simulink model "W3prob2"  (R2020b)
settings: Solver=VariableStepAuto  StartTime=0.0  StopTime=10.0  RelTol=1e-3
settings Model: Creator=deves  LastModifiedBy=deves

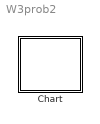
== system W3prob2 ==
  Chart : Stateflow chart  TreatAsAtomicUnit=on

== stateflow chart W3prob2/Chart ==
  state Halt
    s1=RED;
    s2=GREEN;
  state GoToHalt
    s1=YELLOW;
    s2=RED;
  state TrafficStop
    s1=RED;
    s2=GREEN;
  state Go
    s1=GREEN;
    s2=RED;
  state Ready
    s1=RED;
    s2=YELLOW;
  (default) -> Halt
  GoToHalt -> Halt
  Halt -> TrafficStop : after(20,tick)
  Go -> GoToHalt
  TrafficStop -> Ready
  Ready -> Go
